simulink model "sampleModel2432_pp_1_2"  (R2018a)
settings: Solver=VariableStepAuto  StartTime=0.0  StopTime=10.0  RelTol=1e-3
undefined symbols (not defined in the file or in its folder): DiscIntNeverNeededParam, sigbuilder_block
libraries: simulink x302
(part 5 of 7)

== system sampleModel2432_pp_1_2/cfblk202/cfblk11 ==
  cfblk1 : Inport
  Action Port : ActionPort  ActionType=else
  cfblk10 : simulink/Discrete/Tapped Delay  vinit=0.0  samptime=-1  NumDelays=1  DelayOrder=Oldest  includeCurrent=off
  cfblk11 : Delay
  cfblk12 : Delay
  cfblk14 : Delay
  cfblk3 : Delay  DelayLengthSource=Input port
      settings: InputPortMap=u0,p1
  cfblk4 : simulink/Continuous/PID Controller (2DOF)  Controller=PID  TimeDomain=Discrete-time  SampleTime=-1  IntegratorMethod=Forward Euler  FilterMethod=Forward Euler  Form=Parallel  UseFilter=on  ControllerParametersSource=internal  P=1  I=1  D=0  N=100  b=1  c=1  InitialConditionSource=internal  InitialConditionForIntegrator=0  InitialConditionForFilter=0  ExternalReset=none  LimitOutput=off  UpperSaturationLimit=inf  LowerSaturationLimit=-inf  LinearizeAsGain=off  AntiWindupMode=none  Kb=1  TrackingMode=off  Kt=1  PParamMin=[]  PParamMax=[]  IParamMin=[]  IParamMax=[]  DParamMin=[]  DParamMax=[]  NParamMin=[]  NParamMax=[]  bParamMin=[]  bParamMax=[]  cParamMin=[]  cParamMax=[]  KbParamMin=[]  KbParamMax=[]  KtParamMin=[]  KtParamMax=[]  POutMin=[]  POutMax=[]  IOutMin=[]  IOutMax=[]  DOutMin=[]  DOutMax=[]  NOutMin=[]  NOutMax=[]  bOutMin=[]  bOutMax=[]  cOutMin=[]  cOutMax=[]  KbOutMin=[]  KbOutMax=[]  KtOutMin=[]  KtOutMax=[]  IntegratorOutMin=[]  IntegratorOutMax=[]  FilterOutMin=[]  FilterOutMax=[]  SumOutMin=[]  SumOutMax=[]  Sum1OutMin=[]  Sum1OutMax=[]  Sum2OutMin=[]  Sum2OutMax=[]  Sum3OutMin=[]  Sum3OutMax=[]  SumI1OutMin=[]  SumI1OutMax=[]  SumI2OutMin=[]  SumI2OutMax=[]  SumI3OutMin=[]  SumI3OutMax=[]  SumDOutMin=[]  SumDOutMax=[]  SaturationOutMin=[]  SaturationOutMax=[]  IntegratorContinuousStateAttributes=''  IntegratorStateMustResolveToSignalObject=off  IntegratorRTWStateStorageClass=Auto  FilterContinuousStateAttributes=''  FilterStateMustResolveToSignalObject=off  FilterRTWStateStorageClass=Auto  DifferentiatorICPrevScaledInput=0  DifferentiatorOutMin=[]  DifferentiatorOutMax=[]  FilterDiffOutCoefMin=[]  FilterDiffOutCoefMax=[]  SumDenOutMin=[]  SumDenOutMax=[]  SumNumOutMin=[]  SumNumOutMax=[]  ReciprocalOutMin=[]  ReciprocalOutMax=[]  DivideOutMin=[]  DivideOutMax=[]  TunerSelectOption=Transfer Function Based (PID Tuner App)
  cfblk5 : simulink/Continuous/PID Controller (2DOF)  Controller=PID  TimeDomain=Discrete-time  SampleTime=-1  IntegratorMethod=Forward Euler  FilterMethod=Forward Euler  Form=Parallel  UseFilter=on  ControllerParametersSource=internal  P=1  I=1  D=0  N=100  b=1  c=1  InitialConditionSource=internal  InitialConditionForIntegrator=0  InitialConditionForFilter=0  ExternalReset=none  LimitOutput=off  UpperSaturationLimit=inf  LowerSaturationLimit=-inf  LinearizeAsGain=off  AntiWindupMode=none  Kb=1  TrackingMode=off  Kt=1  PParamMin=[]  PParamMax=[]  IParamMin=[]  IParamMax=[]  DParamMin=[]  DParamMax=[]  NParamMin=[]  NParamMax=[]  bParamMin=[]  bParamMax=[]  cParamMin=[]  cParamMax=[]  KbParamMin=[]  KbParamMax=[]  KtParamMin=[]  KtParamMax=[]  POutMin=[]  POutMax=[]  IOutMin=[]  IOutMax=[]  DOutMin=[]  DOutMax=[]  NOutMin=[]  NOutMax=[]  bOutMin=[]  bOutMax=[]  cOutMin=[]  cOutMax=[]  KbOutMin=[]  KbOutMax=[]  KtOutMin=[]  KtOutMax=[]  IntegratorOutMin=[]  IntegratorOutMax=[]  FilterOutMin=[]  FilterOutMax=[]  SumOutMin=[]  SumOutMax=[]  Sum1OutMin=[]  Sum1OutMax=[]  Sum2OutMin=[]  Sum2OutMax=[]  Sum3OutMin=[]  Sum3OutMax=[]  SumI1OutMin=[]  SumI1OutMax=[]  SumI2OutMin=[]  SumI2OutMax=[]  SumI3OutMin=[]  SumI3OutMax=[]  SumDOutMin=[]  SumDOutMax=[]  SaturationOutMin=[]  SaturationOutMax=[]  IntegratorContinuousStateAttributes=''  IntegratorStateMustResolveToSignalObject=off  IntegratorRTWStateStorageClass=Auto  FilterContinuousStateAttributes=''  FilterStateMustResolveToSignalObject=off  FilterRTWStateStorageClass=Auto  DifferentiatorICPrevScaledInput=0  DifferentiatorOutMin=[]  DifferentiatorOutMax=[]  FilterDiffOutCoefMin=[]  FilterDiffOutCoefMax=[]  SumDenOutMin=[]  SumDenOutMax=[]  SumNumOutMin=[]  SumNumOutMax=[]  ReciprocalOutMin=[]  ReciprocalOutMax=[]  DivideOutMin=[]  DivideOutMax=[]  TunerSelectOption=Transfer Function Based (PID Tuner App)
  cfblk6 : simulink/Continuous/PID Controller (2DOF)  Controller=PID  TimeDomain=Discrete-time  SampleTime=-1  IntegratorMethod=Forward Euler  FilterMethod=Forward Euler  Form=Parallel  UseFilter=on  ControllerParametersSource=internal  P=1  I=1  D=0  N=100  b=1  c=1  InitialConditionSource=internal  InitialConditionForIntegrator=0  InitialConditionForFilter=0  ExternalReset=none  LimitOutput=off  UpperSaturationLimit=inf  LowerSaturationLimit=-inf  LinearizeAsGain=off  AntiWindupMode=none  Kb=1  TrackingMode=off  Kt=1  PParamMin=[]  PParamMax=[]  IParamMin=[]  IParamMax=[]  DParamMin=[]  DParamMax=[]  NParamMin=[]  NParamMax=[]  bParamMin=[]  bParamMax=[]  cParamMin=[]  cParamMax=[]  KbParamMin=[]  KbParamMax=[]  KtParamMin=[]  KtParamMax=[]  POutMin=[]  POutMax=[]  IOutMin=[]  IOutMax=[]  DOutMin=[]  DOutMax=[]  NOutMin=[]  NOutMax=[]  bOutMin=[]  bOutMax=[]  cOutMin=[]  cOutMax=[]  KbOutMin=[]  KbOutMax=[]  KtOutMin=[]  KtOutMax=[]  IntegratorOutMin=[]  IntegratorOutMax=[]  FilterOutMin=[]  FilterOutMax=[]  SumOutMin=[]  SumOutMax=[]  Sum1OutMin=[]  Sum1OutMax=[]  Sum2OutMin=[]  Sum2OutMax=[]  Sum3OutMin=[]  Sum3OutMax=[]  SumI1OutMin=[]  SumI1OutMax=[]  SumI2OutMin=[]  SumI2OutMax=[]  SumI3OutMin=[]  SumI3OutMax=[]  SumDOutMin=[]  SumDOutMax=[]  SaturationOutMin=[]  SaturationOutMax=[]  IntegratorContinuousStateAttributes=''  IntegratorStateMustResolveToSignalObject=off  IntegratorRTWStateStorageClass=Auto  FilterContinuousStateAttributes=''  FilterStateMustResolveToSignalObject=off  FilterRTWStateStorageClass=Auto  DifferentiatorICPrevScaledInput=0  DifferentiatorOutMin=[]  DifferentiatorOutMax=[]  FilterDiffOutCoefMin=[]  FilterDiffOutCoefMax=[]  SumDenOutMin=[]  SumDenOutMax=[]  SumNumOutMin=[]  SumNumOutMax=[]  ReciprocalOutMin=[]  ReciprocalOutMax=[]  DivideOutMin=[]  DivideOutMax=[]  TunerSelectOption=Transfer Function Based (PID Tuner App)
  cfblk7 : DiscreteTransferFcn
  cfblk8 : DiscreteFilter
  cfblk9 : simulink/Discrete/Transfer Fcn Real Zero  ZeroZ=0.75  ICPrevInput=0.0  DoSatur=off
      settings: SourceProductName=Simulink  SourceProductBaseCode=SL
  cyemi_{239..253} (15 alike) : DataTypeConversion  OutDataTypeStr=double
  cfblk2 : Outport
  cfblk13 : Outport  Port=2
  wires:
  cfblk7/1 -> cyemi_244/1, cyemi_246/1
  cfblk9/1 -> cyemi_241/1, cyemi_242/1
  cfblk10/1 -> cyemi_240/1, cyemi_245/1, cyemi_252/1
  cfblk5/1 -> cfblk2/1, cyemi_253/1
  cfblk6/1 -> cfblk13/1
  cyemi_239/1 -> cfblk10/1
  cfblk1/1 -> cyemi_239/1
  cyemi_240/1 -> cfblk11/1
  cyemi_241/1 -> cfblk12/1
  cyemi_242/1 -> cfblk14/1
  cyemi_243/1 -> cfblk3/1
  cfblk8/1 -> cyemi_243/1
  cyemi_244/1 -> cfblk3/2
  cyemi_245/1 -> cfblk4/1
  cyemi_246/1 -> cfblk4/2
  cyemi_247/1 -> cfblk5/1
  cfblk3/1 -> cyemi_247/1
  cyemi_248/1 -> cfblk5/2
  cfblk14/1 -> cyemi_248/1
  cyemi_249/1 -> cfblk6/1
  cfblk4/1 -> cyemi_249/1
  cyemi_250/1 -> cfblk6/2
  cfblk12/1 -> cyemi_250/1
  cyemi_251/1 -> cfblk7/1
  cfblk11/1 -> cyemi_251/1
  cyemi_252/1 -> cfblk8/1
  cyemi_253/1 -> cfblk9/1

== system sampleModel2432_pp_1_2/cfblk202/cfblk12 ==
  cfblk1 : Inport
  cfblk15 : Inport  Port=2
  Action Port : ActionPort  ActionType=then
  cfblk12 : DiscreteStateSpace  SampleTime=-1
  cfblk14 : DiscreteTransferFcn
  cfblk17 : Delay
  cfblk4 : Delay
  cfblk5 : DiscreteTransferFcn
  cfblk6 : simulink/Discrete/Transfer Fcn Lead or Lag  PoleZ=0.95  ZeroZ=0.75  ICPrevOutput=0.0  ICPrevInput=0.0  DoSatur=off
      settings: SourceProductName=Simulink  SourceProductBaseCode=SL
  cfblk8 : Delay
  cyemi_{256..269} (14 alike) : DataTypeConversion  OutDataTypeStr=double
  cfblk2 : Outport
  cfblk16 : Outport  Port=2
  wires:
  cfblk4/1 -> cyemi_260/1, cyemi_265/1
  cfblk6/1 -> cyemi_256/1
  cfblk15/1 -> cyemi_258/1
  cyemi_259/1 -> cfblk12/1
  cyemi_261/1 -> cfblk14/1
  cfblk8/1 -> cyemi_261/1
  cyemi_262/1 -> cfblk17/1
  cfblk12/1 -> cyemi_262/1
  cfblk17/1 -> cyemi_263/1
  cyemi_264/1 -> cfblk4/1
  cyemi_265/1 -> cfblk5/1
  cyemi_266/1 -> cfblk6/1
  cfblk14/1 -> cyemi_266/1
  cfblk1/1 -> cyemi_267/1
  cyemi_268/1 -> cfblk8/1
  cfblk5/1 -> cyemi_269/1
  cyemi_260/1 -> cfblk2/1
  cyemi_263/1 -> cyemi_268/1
  cyemi_258/1 -> cyemi_264/1
  cyemi_269/1 -> cyemi_257/1
  cyemi_267/1 -> cfblk16/1
  cyemi_256/1 -> cyemi_259/1

== system sampleModel2432_pp_1_2/cfblk202/cfblk13 ==
  cfblk1 : Inport
  cfblk7 : Inport  Port=2
  Action Port : ActionPort  ActionType=else
  cfblk3 : simulink/Discrete/Transfer Fcn Real Zero  ZeroZ=0.75  ICPrevInput=0.0  DoSatur=off
      settings: SourceProductName=Simulink  SourceProductBaseCode=SL
  cfblk4 : Delay  ShowEnablePort=on
      settings: InputPortMap=u0,e6
  cfblk5 : Delay  DelayLengthSource=Input port
      settings: InputPortMap=u0,p1
  cfblk6 : simulink/Discrete/Tapped Delay  vinit=0.0  samptime=-1  NumDelays=1  DelayOrder=Oldest  includeCurrent=off
  cyemi_{272..277} (6 alike) : DataTypeConversion  OutDataTypeStr=double
  cfblk2 : Outport
  wires:
  cfblk4/1 -> cfblk2/1
  cfblk6/1 -> cyemi_274/1, cyemi_276/1
  cyemi_272/1 -> cfblk3/1
  cfblk5/1 -> cyemi_272/1
  cyemi_273/1 -> cfblk4/1
  cfblk3/1 -> cyemi_273/1
  cyemi_274/1 -> cfblk4/2
  cyemi_275/1 -> cfblk5/1
  cfblk7/1 -> cyemi_275/1
  cyemi_276/1 -> cfblk5/2
  cyemi_277/1 -> cfblk6/1
  cfblk1/1 -> cyemi_277/1

== system sampleModel2432_pp_1_2/cfblk204/cfblk13 ==
  cfblk1 : Inport
  cfblk11 : Inport  Port=2
  Action Port : ActionPort  ActionType=then
  cfblk3 : simulink/Discrete/Transfer Fcn Real Zero  ZeroZ=0.75  ICPrevInput=0.0  DoSatur=off
      settings: SourceProductName=Simulink  SourceProductBaseCode=SL
  cfblk4 : simulink/Discrete/Transfer Fcn First Order  PoleZ=0.95  ICPrevOutput=0.0  DoSatur=off
      settings: SourceProductName=Simulink
  cfblk8 : DiscreteStateSpace  SampleTime=-1
  cfblk9 : Delay
  cyemi_{310..317} (8 alike) : DataTypeConversion  OutDataTypeStr=double
  cfblk2 : Outport
  cfblk12 : Outport  Port=2
  wires:
  cfblk9/1 -> cfblk12/1
  cfblk4/1 -> cfblk2/1
  cfblk1/1 -> cyemi_310/1
  cyemi_311/1 -> cfblk3/1
  cyemi_312/1 -> cfblk4/1
  cfblk11/1 -> cyemi_312/1
  cyemi_316/1 -> cfblk8/1
  cfblk3/1 -> cyemi_316/1
  cyemi_317/1 -> cfblk9/1
  cfblk8/1 -> cyemi_317/1
  cyemi_313/1 -> cyemi_311/1
  cyemi_315/1 -> cyemi_314/1
  cyemi_314/1 -> cyemi_313/1
  cyemi_310/1 -> cyemi_315/1

== system sampleModel2432_pp_1_2/cfblk204/cfblk14 ==
  cfblk1 : Inport
  cfblk9 : Inport  Port=2
  Action Port : ActionPort  ActionType=else
  cfblk3 : DiscreteZeroPole  Poles=[0 0.5]  Gain=1  SampleTime=-1
  cfblk4 : UnitDelay  SampleTime=-1
  cfblk5 : simulink/Discrete/Tapped Delay  vinit=0.0  samptime=-1  NumDelays=1  DelayOrder=Oldest  includeCurrent=off
  cfblk6 : UnitDelay  SampleTime=-1
  cfblk7 : DiscreteZeroPole  Poles=[0 0.5]  Gain=1  SampleTime=-1
  cfblk8 : simulink/Discrete/Transfer Fcn First Order  PoleZ=0.95  ICPrevOutput=0.0  DoSatur=off
      settings: SourceProductName=Simulink
  cyemi_{320..325} (6 alike) : DataTypeConversion  OutDataTypeStr=double
  cfblk2 : Outport
  cfblk10 : Outport  Port=2
  cfblk11 : Outport  Port=3
  cfblk12 : Outport  Port=4
  wires:
  cfblk7/1 -> cfblk10/1
  cfblk8/1 -> cfblk12/1
  cfblk3/1 -> cfblk2/1, cyemi_324/1
  cfblk5/1 -> cfblk11/1, cyemi_320/1
  cyemi_320/1 -> cfblk3/1
  cyemi_321/1 -> cfblk4/1
  cfblk1/1 -> cyemi_321/1
  cyemi_322/1 -> cfblk5/1
  cfblk6/1 -> cyemi_322/1
  cyemi_323/1 -> cfblk6/1
  cfblk4/1 -> cyemi_323/1
  cyemi_324/1 -> cfblk7/1
  cyemi_325/1 -> cfblk8/1
  cfblk9/1 -> cyemi_325/1

== system sampleModel2432_pp_1_2/cfblk206/cfblk11 ==
  cfblk1 : Inport
  cfblk8 : Inport  Port=2
  cfblk9 : Inport  Port=3
  Action Port : ActionPort  ActionType=then
  cfblk3 : simulink/Discrete/Difference  ICPrevInput=0.0  OutMin=[]  OutMax=[]  OutDataTypeStr=Inherit: Inherit via back propagation  OutDataType=fixdt(1, 16)  OutScaling=2^-10  DoSatur=off
  cfblk5 : simulink/Discrete/Difference  ICPrevInput=0.0  OutMin=[]  OutMax=[]  OutDataTypeStr=Inherit: Inherit via back propagation  OutDataType=fixdt(1, 16)  OutScaling=2^-10  DoSatur=off
  cfblk6 : simulink/Discrete/Transfer Fcn Real Zero  ZeroZ=0.75  ICPrevInput=0.0  DoSatur=off
      settings: SourceProductName=Simulink  SourceProductBaseCode=SL
  cyemi_{344..348} (5 alike) : DataTypeConversion  OutDataTypeStr=double
  cfblk2 : Outport
  cfblk10 : Outport  Port=2
  wires:
  cfblk9/1 -> cfblk10/1
  cyemi_344/1 -> cfblk3/1
  cfblk6/1 -> cyemi_344/1
  cfblk5/1 -> cyemi_345/1
  cyemi_346/1 -> cfblk5/1
  cfblk8/1 -> cyemi_346/1
  cyemi_347/1 -> cfblk6/1
  cfblk1/1 -> cyemi_347/1
  cyemi_345/1 -> cyemi_348/1
  cyemi_348/1 -> cfblk2/1

== system sampleModel2432_pp_1_2/cfblk206/cfblk12 ==
  cfblk1 : Inport
  cfblk13 : Inport  Port=2
  cfblk14 : Inport  Port=3
  Action Port : ActionPort  ActionType=else
  cfblk10 : simulink/Discrete/Difference  ICPrevInput=0.0  OutMin=[]  OutMax=[]  OutDataTypeStr=Inherit: Inherit via back propagation  OutDataType=fixdt(1, 16)  OutScaling=2^-10  DoSatur=off
  cfblk11 : DiscreteZeroPole  Poles=[0 0.5]  Gain=1  SampleTime=-1
  cfblk12 : UnitDelay  SampleTime=-1
  cfblk16 : Delay
  cfblk3 : DiscreteZeroPole  Poles=[0 0.5]  Gain=1  SampleTime=-1
  cfblk4 : DiscreteFilter
  cfblk5 : DiscreteFilter
  cfblk6 : DiscreteStateSpace  SampleTime=-1
  cfblk7 : DiscreteStateSpace  SampleTime=-1
  cfblk8 : DiscreteTransferFcn
  cfblk9 : DiscreteFilter
  cyemi_{352..362} (11 alike) : DataTypeConversion  OutDataTypeStr=double
  cfblk2 : Outport
  cfblk15 : Outport  Port=2
  wires:
  cfblk10/1 -> cfblk15/1
  cfblk6/1 -> cfblk2/1
  cyemi_352/1 -> cfblk10/1
  cfblk5/1 -> cyemi_352/1
  cyemi_353/1 -> cfblk11/1
  cfblk7/1 -> cyemi_353/1
  cyemi_354/1 -> cfblk12/1
  cfblk13/1 -> cyemi_354/1
  cyemi_355/1 -> cfblk16/1
  cfblk11/1 -> cyemi_355/1
  cyemi_356/1 -> cfblk3/1
  cfblk14/1 -> cyemi_356/1
  cyemi_357/1 -> cfblk4/1
  cfblk16/1 -> cyemi_357/1
  cyemi_358/1 -> cfblk5/1
  cfblk1/1 -> cyemi_358/1
  cyemi_359/1 -> cfblk6/1
  cfblk8/1 -> cyemi_359/1
  cyemi_360/1 -> cfblk7/1
  cfblk9/1 -> cyemi_360/1
  cyemi_361/1 -> cfblk8/1
  cfblk3/1 -> cyemi_361/1
  cyemi_362/1 -> cfblk9/1
  cfblk4/1 -> cyemi_362/1

== system sampleModel2432_pp_1_2/cfblk210/cfblk10 ==
  cfblk1 : Inport
  Action Port : ActionPort  ActionType=then
  cfblk3 : simulink/Discrete/Transfer Fcn First Order  PoleZ=0.95  ICPrevOutput=0.0  DoSatur=off
      settings: SourceProductName=Simulink
  cfblk4 : DiscreteTransferFcn
  cfblk5 : simulink/Discrete/Transfer Fcn Lead or Lag  PoleZ=0.95  ZeroZ=0.75  ICPrevOutput=0.0  ICPrevInput=0.0  DoSatur=off
      settings: SourceProductName=Simulink  SourceProductBaseCode=SL
  cfblk9 : Delay
  cyemi_{399..404} (6 alike) : DataTypeConversion  OutDataTypeStr=double
  cfblk2 : Outport
  cfblk7 : Outport  Port=2
  cfblk8 : Outport  Port=3
  wires:
  cfblk5/1 -> cfblk8/1, cyemi_404/1
  cfblk4/1 -> cfblk2/1, cyemi_401/1
  cfblk1/1 -> cfblk7/1, cyemi_403/1
  cyemi_399/1 -> cfblk3/1
  cyemi_400/1 -> cfblk4/1
  cfblk3/1 -> cyemi_400/1
  cyemi_401/1 -> cfblk5/1
  cfblk9/1 -> cyemi_402/1
  cyemi_404/1 -> cfblk9/1
  cyemi_402/1 -> cyemi_399/1

== system sampleModel2432_pp_1_2/cfblk210/cfblk11 ==
  cfblk1 : Inport
  cfblk12 : Inport  Port=2
  Action Port : ActionPort  ActionType=else
  cfblk10 : DiscreteStateSpace  SampleTime=-1
  cfblk11 : DiscreteStateSpace  SampleTime=-1
  cfblk15 : Delay
  cfblk3 : simulink/Continuous/PID Controller (2DOF)  Controller=PID  TimeDomain=Discrete-time  SampleTime=-1  IntegratorMethod=Forward Euler  FilterMethod=Forward Euler  Form=Parallel  UseFilter=on  ControllerParametersSource=internal  P=1  I=1  D=0  N=100  b=1  c=1  InitialConditionSource=internal  InitialConditionForIntegrator=0  InitialConditionForFilter=0  ExternalReset=none  LimitOutput=off  UpperSaturationLimit=inf  LowerSaturationLimit=-inf  LinearizeAsGain=off  AntiWindupMode=none  Kb=1  TrackingMode=off  Kt=1  PParamMin=[]  PParamMax=[]  IParamMin=[]  IParamMax=[]  DParamMin=[]  DParamMax=[]  NParamMin=[]  NParamMax=[]  bParamMin=[]  bParamMax=[]  cParamMin=[]  cParamMax=[]  KbParamMin=[]  KbParamMax=[]  KtParamMin=[]  KtParamMax=[]  POutMin=[]  POutMax=[]  IOutMin=[]  IOutMax=[]  DOutMin=[]  DOutMax=[]  NOutMin=[]  NOutMax=[]  bOutMin=[]  bOutMax=[]  cOutMin=[]  cOutMax=[]  KbOutMin=[]  KbOutMax=[]  KtOutMin=[]  KtOutMax=[]  IntegratorOutMin=[]  IntegratorOutMax=[]  FilterOutMin=[]  FilterOutMax=[]  SumOutMin=[]  SumOutMax=[]  Sum1OutMin=[]  Sum1OutMax=[]  Sum2OutMin=[]  Sum2OutMax=[]  Sum3OutMin=[]  Sum3OutMax=[]  SumI1OutMin=[]  SumI1OutMax=[]  SumI2OutMin=[]  SumI2OutMax=[]  SumI3OutMin=[]  SumI3OutMax=[]  SumDOutMin=[]  SumDOutMax=[]  SaturationOutMin=[]  SaturationOutMax=[]  IntegratorContinuousStateAttributes=''  IntegratorStateMustResolveToSignalObject=off  IntegratorRTWStateStorageClass=Auto  FilterContinuousStateAttributes=''  FilterStateMustResolveToSignalObject=off  FilterRTWStateStorageClass=Auto  DifferentiatorICPrevScaledInput=0  DifferentiatorOutMin=[]  DifferentiatorOutMax=[]  FilterDiffOutCoefMin=[]  FilterDiffOutCoefMax=[]  SumDenOutMin=[]  SumDenOutMax=[]  SumNumOutMin=[]  SumNumOutMax=[]  ReciprocalOutMin=[]  ReciprocalOutMax=[]  DivideOutMin=[]  DivideOutMax=[]  TunerSelectOption=Transfer Function Based (PID Tuner App)
  cfblk4 : DiscreteZeroPole  Poles=[0 0.5]  Gain=1  SampleTime=-1
  cfblk5 : simulink/Discrete/Transfer Fcn Real Zero  ZeroZ=0.75  ICPrevInput=0.0  DoSatur=off
      settings: SourceProductName=Simulink  SourceProductBaseCode=SL
  cfblk6 : Delay  ShowEnablePort=on
      settings: InputPortMap=u0,e6
  cfblk7 : simulink/Continuous/PID Controller (2DOF)  Controller=PID  TimeDomain=Discrete-time  SampleTime=-1  IntegratorMethod=Forward Euler  FilterMethod=Forward Euler  Form=Parallel  UseFilter=on  ControllerParametersSource=internal  P=1  I=1  D=0  N=100  b=1  c=1  InitialConditionSource=internal  InitialConditionForIntegrator=0  InitialConditionForFilter=0  ExternalReset=none  LimitOutput=off  UpperSaturationLimit=inf  LowerSaturationLimit=-inf  LinearizeAsGain=off  AntiWindupMode=none  Kb=1  TrackingMode=off  Kt=1  PParamMin=[]  PParamMax=[]  IParamMin=[]  IParamMax=[]  DParamMin=[]  DParamMax=[]  NParamMin=[]  NParamMax=[]  bParamMin=[]  bParamMax=[]  cParamMin=[]  cParamMax=[]  KbParamMin=[]  KbParamMax=[]  KtParamMin=[]  KtParamMax=[]  POutMin=[]  POutMax=[]  IOutMin=[]  IOutMax=[]  DOutMin=[]  DOutMax=[]  NOutMin=[]  NOutMax=[]  bOutMin=[]  bOutMax=[]  cOutMin=[]  cOutMax=[]  KbOutMin=[]  KbOutMax=[]  KtOutMin=[]  KtOutMax=[]  IntegratorOutMin=[]  IntegratorOutMax=[]  FilterOutMin=[]  FilterOutMax=[]  SumOutMin=[]  SumOutMax=[]  Sum1OutMin=[]  Sum1OutMax=[]  Sum2OutMin=[]  Sum2OutMax=[]  Sum3OutMin=[]  Sum3OutMax=[]  SumI1OutMin=[]  SumI1OutMax=[]  SumI2OutMin=[]  SumI2OutMax=[]  SumI3OutMin=[]  SumI3OutMax=[]  SumDOutMin=[]  SumDOutMax=[]  SaturationOutMin=[]  SaturationOutMax=[]  IntegratorContinuousStateAttributes=''  IntegratorStateMustResolveToSignalObject=off  IntegratorRTWStateStorageClass=Auto  FilterContinuousStateAttributes=''  FilterStateMustResolveToSignalObject=off  FilterRTWStateStorageClass=Auto  DifferentiatorICPrevScaledInput=0  DifferentiatorOutMin=[]  DifferentiatorOutMax=[]  FilterDiffOutCoefMin=[]  FilterDiffOutCoefMax=[]  SumDenOutMin=[]  SumDenOutMax=[]  SumNumOutMin=[]  SumNumOutMax=[]  ReciprocalOutMin=[]  ReciprocalOutMax=[]  DivideOutMin=[]  DivideOutMax=[]  TunerSelectOption=Transfer Function Based (PID Tuner App)
  cfblk8 : DiscreteFir
  cfblk9 : DiscreteZeroPole  Poles=[0 0.5]  Gain=1  SampleTime=-1
  cyemi_{407..419} (13 alike) : DataTypeConversion  OutDataTypeStr=double
  cfblk2 : Outport
  cfblk13 : Outport  Port=2
  cfblk14 : Outport  Port=3
  wires:
  cfblk8/1 -> cfblk2/1, cyemi_408/1
  cfblk11/1 -> cyemi_407/1, cyemi_414/1
  cfblk7/1 -> cfblk13/1
  cfblk3/1 -> cfblk14/1, cyemi_415/1
  cyemi_407/1 -> cfblk10/1
  cyemi_408/1 -> cfblk11/1
  cyemi_409/1 -> cfblk15/1
  cfblk10/1 -> cyemi_409/1
  cyemi_410/1 -> cfblk3/1
  cfblk12/1 -> cyemi_410/1
  cyemi_411/1 -> cfblk3/2
  cfblk4/1 -> cyemi_411/1
  cyemi_412/1 -> cfblk4/1
  cfblk9/1 -> cyemi_412/1
  cyemi_413/1 -> cfblk5/1
  cfblk15/1 -> cyemi_413/1
  cyemi_414/1 -> cfblk6/1
  cyemi_415/1 -> cfblk6/2
  cyemi_416/1 -> cfblk7/1
  cfblk6/1 -> cyemi_416/1, cyemi_417/1
  cyemi_417/1 -> cfblk7/2
  cyemi_418/1 -> cfblk8/1
  cfblk5/1 -> cyemi_418/1
  cyemi_419/1 -> cfblk9/1
  cfblk1/1 -> cyemi_419/1

== system sampleModel2432_pp_1_2/cfblk218/cfblk18 ==
  cfblk1 : Inport
  cfblk11 : Inport  Port=2
  Action Port : ActionPort  ActionType=then
  cfblk10 : simulink/Discrete/Transfer Fcn First Order  PoleZ=0.95  ICPrevOutput=0.0  DoSatur=off
      settings: SourceProductName=Simulink
  cfblk5 : DiscreteStateSpace  SampleTime=-1
  cfblk6 : Delay
  cfblk7 : simulink/Discrete/Transfer Fcn Lead or Lag  PoleZ=0.95  ZeroZ=0.75  ICPrevOutput=0.0  ICPrevInput=0.0  DoSatur=off
      settings: SourceProductName=Simulink  SourceProductBaseCode=SL
  cfblk9 : DiscreteFir
  cyemi_{505..512} (8 alike) : DataTypeConversion  OutDataTypeStr=double
  cfblk2 : Outport
  cfblk12 : Outport  Port=2
  cfblk13 : Outport  Port=3
  wires:
  cfblk7/1 -> cfblk13/1
  cfblk1/1 -> cfblk12/1
  cfblk11/1 -> cyemi_510/1, cyemi_511/1
  cyemi_505/1 -> cfblk10/1
  cfblk9/1 -> cyemi_505/1
  cfblk5/1 -> cyemi_506/1
  cfblk10/1 -> cyemi_507/1
  cyemi_508/1 -> cfblk5/1
  cfblk6/1 -> cyemi_508/1
  cyemi_509/1 -> cfblk6/1
  cyemi_510/1 -> cfblk7/1
  cyemi_512/1 -> cfblk9/1
  cyemi_507/1 -> cyemi_509/1
  cyemi_511/1 -> cyemi_512/1
  cyemi_506/1 -> cfblk2/1

== system sampleModel2432_pp_1_2/cfblk218/cfblk19 ==
  cfblk1 : Inport
  cfblk10 : Inport  Port=2
  Action Port : ActionPort  ActionType=else
  cfblk11 : Delay
  cfblk3 : simulink/Discrete/Tapped Delay  vinit=0.0  samptime=-1  NumDelays=1  DelayOrder=Oldest  includeCurrent=off
  cfblk4 : Delay
  cfblk5 : Delay  ShowEnablePort=on
      settings: InputPortMap=u0,e6
  cfblk6 : DiscreteZeroPole  Poles=[0 0.5]  Gain=1  SampleTime=-1
  cfblk7 : simulink/Continuous/PID Controller (2DOF)  Controller=PID  TimeDomain=Discrete-time  SampleTime=-1  IntegratorMethod=Forward Euler  FilterMethod=Forward Euler  Form=Parallel  UseFilter=on  ControllerParametersSource=internal  P=1  I=1  D=0  N=100  b=1  c=1  InitialConditionSource=internal  InitialConditionForIntegrator=0  InitialConditionForFilter=0  ExternalReset=none  LimitOutput=off  UpperSaturationLimit=inf  LowerSaturationLimit=-inf  LinearizeAsGain=off  AntiWindupMode=none  Kb=1  TrackingMode=off  Kt=1  PParamMin=[]  PParamMax=[]  IParamMin=[]  IParamMax=[]  DParamMin=[]  DParamMax=[]  NParamMin=[]  NParamMax=[]  bParamMin=[]  bParamMax=[]  cParamMin=[]  cParamMax=[]  KbParamMin=[]  KbParamMax=[]  KtParamMin=[]  KtParamMax=[]  POutMin=[]  POutMax=[]  IOutMin=[]  IOutMax=[]  DOutMin=[]  DOutMax=[]  NOutMin=[]  NOutMax=[]  bOutMin=[]  bOutMax=[]  cOutMin=[]  cOutMax=[]  KbOutMin=[]  KbOutMax=[]  KtOutMin=[]  KtOutMax=[]  IntegratorOutMin=[]  IntegratorOutMax=[]  FilterOutMin=[]  FilterOutMax=[]  SumOutMin=[]  SumOutMax=[]  Sum1OutMin=[]  Sum1OutMax=[]  Sum2OutMin=[]  Sum2OutMax=[]  Sum3OutMin=[]  Sum3OutMax=[]  SumI1OutMin=[]  SumI1OutMax=[]  SumI2OutMin=[]  SumI2OutMax=[]  SumI3OutMin=[]  SumI3OutMax=[]  SumDOutMin=[]  SumDOutMax=[]  SaturationOutMin=[]  SaturationOutMax=[]  IntegratorContinuousStateAttributes=''  IntegratorStateMustResolveToSignalObject=off  IntegratorRTWStateStorageClass=Auto  FilterContinuousStateAttributes=''  FilterStateMustResolveToSignalObject=off  FilterRTWStateStorageClass=Auto  DifferentiatorICPrevScaledInput=0  DifferentiatorOutMin=[]  DifferentiatorOutMax=[]  FilterDiffOutCoefMin=[]  FilterDiffOutCoefMax=[]  SumDenOutMin=[]  SumDenOutMax=[]  SumNumOutMin=[]  SumNumOutMax=[]  ReciprocalOutMin=[]  ReciprocalOutMax=[]  DivideOutMin=[]  DivideOutMax=[]  TunerSelectOption=Transfer Function Based (PID Tuner App)
  cfblk8 : simulink/Discrete/Difference  ICPrevInput=0.0  OutMin=[]  OutMax=[]  OutDataTypeStr=Inherit: Inherit via back propagation  OutDataType=fixdt(1, 16)  OutScaling=2^-10  DoSatur=off
  cfblk9 : simulink/Discrete/Difference  ICPrevInput=0.0  OutMin=[]  OutMax=[]  OutDataTypeStr=Inherit: Inherit via back propagation  OutDataType=fixdt(1, 16)  OutScaling=2^-10  DoSatur=off
  cyemi_{515..524} (10 alike) : DataTypeConversion  OutDataTypeStr=double
  cfblk2 : Outport
  wires:
  cfblk6/1 -> cfblk2/1
  cfblk10/1 -> cyemi_520/1, cyemi_522/1
  cyemi_515/1 -> cfblk11/1
  cfblk4/1 -> cyemi_515/1
  cyemi_516/1 -> cfblk3/1
  cfblk8/1 -> cyemi_516/1
  cyemi_517/1 -> cfblk4/1
  cfblk5/1 -> cyemi_517/1
  cyemi_518/1 -> cfblk5/1
  cfblk11/1 -> cyemi_518/1
  cyemi_519/1 -> cfblk5/2
  cfblk3/1 -> cyemi_519/1
  cyemi_520/1 -> cfblk6/1
  cyemi_521/1 -> cfblk7/1
  cfblk1/1 -> cyemi_521/1
  cyemi_522/1 -> cfblk7/2
  cyemi_523/1 -> cfblk8/1
  cfblk9/1 -> cyemi_523/1
  cyemi_524/1 -> cfblk9/1
  cfblk7/1 -> cyemi_524/1

== system sampleModel2432_pp_1_2/cfblk218/cfblk20 ==
  cfblk1 : Inport
  cfblk10 : Inport  Port=2
  Action Port : ActionPort  ActionType=then
  cfblk3 : DiscreteIntegrator  SampleTime=-1  ICPrevOutput=DiscIntNeverNeededParam  ICPrevScaledInput=DiscIntNeverNeededParam
  cfblk4 : simulink/Discrete/Transfer Fcn Real Zero  ZeroZ=0.75  ICPrevInput=0.0  DoSatur=off
      settings: SourceProductName=Simulink  SourceProductBaseCode=SL
  cfblk6 : DiscreteTransferFcn
  cfblk7 : DiscreteIntegrator  SampleTime=-1  ICPrevOutput=DiscIntNeverNeededParam  ICPrevScaledInput=DiscIntNeverNeededParam
  cfblk9 : DiscreteIntegrator  SampleTime=-1  ICPrevOutput=DiscIntNeverNeededParam  ICPrevScaledInput=DiscIntNeverNeededParam
  cyemi_{527..533} (7 alike) : DataTypeConversion  OutDataTypeStr=double
  cfblk2 : Outport
  cfblk11 : Outport  Port=2
  cfblk12 : Outport  Port=3
  cfblk13 : Outport  Port=4
  cfblk14 : Outport  Port=5
  cfblk15 : Outport  Port=6
  wires:
  cfblk9/1 -> cfblk13/1
  cfblk4/1 -> cfblk14/1
  cfblk6/1 -> cfblk12/1, cfblk2/1, cyemi_529/1
  cfblk3/1 -> cfblk15/1, cyemi_533/1
  cyemi_527/1 -> cfblk3/1
  cfblk10/1 -> cyemi_527/1
  cyemi_528/1 -> cfblk4/1
  cfblk7/1 -> cyemi_528/1
  cyemi_530/1 -> cfblk6/1
  cfblk1/1 -> cyemi_530/1
  cyemi_531/1 -> cfblk7/1
  cyemi_533/1 -> cfblk9/1
  cyemi_532/1 -> cyemi_531/1
  cyemi_529/1 -> cyemi_532/1, cfblk11/1

== system sampleModel2432_pp_1_2/cfblk218/cfblk21 ==
  cfblk1 : Inport
  cfblk6 : Inport  Port=2
  Action Port : ActionPort  ActionType=else
  cfblk3 : simulink/Continuous/PID Controller (2DOF)  Controller=PID  TimeDomain=Discrete-time  SampleTime=-1  IntegratorMethod=Forward Euler  FilterMethod=Forward Euler  Form=Parallel  UseFilter=on  ControllerParametersSource=internal  P=1  I=1  D=0  N=100  b=1  c=1  InitialConditionSource=internal  InitialConditionForIntegrator=0  InitialConditionForFilter=0  ExternalReset=none  LimitOutput=off  UpperSaturationLimit=inf  LowerSaturationLimit=-inf  LinearizeAsGain=off  AntiWindupMode=none  Kb=1  TrackingMode=off  Kt=1  PParamMin=[]  PParamMax=[]  IParamMin=[]  IParamMax=[]  DParamMin=[]  DParamMax=[]  NParamMin=[]  NParamMax=[]  bParamMin=[]  bParamMax=[]  cParamMin=[]  cParamMax=[]  KbParamMin=[]  KbParamMax=[]  KtParamMin=[]  KtParamMax=[]  POutMin=[]  POutMax=[]  IOutMin=[]  IOutMax=[]  DOutMin=[]  DOutMax=[]  NOutMin=[]  NOutMax=[]  bOutMin=[]  bOutMax=[]  cOutMin=[]  cOutMax=[]  KbOutMin=[]  KbOutMax=[]  KtOutMin=[]  KtOutMax=[]  IntegratorOutMin=[]  IntegratorOutMax=[]  FilterOutMin=[]  FilterOutMax=[]  SumOutMin=[]  SumOutMax=[]  Sum1OutMin=[]  Sum1OutMax=[]  Sum2OutMin=[]  Sum2OutMax=[]  Sum3OutMin=[]  Sum3OutMax=[]  SumI1OutMin=[]  SumI1OutMax=[]  SumI2OutMin=[]  SumI2OutMax=[]  SumI3OutMin=[]  SumI3OutMax=[]  SumDOutMin=[]  SumDOutMax=[]  SaturationOutMin=[]  SaturationOutMax=[]  IntegratorContinuousStateAttributes=''  IntegratorStateMustResolveToSignalObject=off  IntegratorRTWStateStorageClass=Auto  FilterContinuousStateAttributes=''  FilterStateMustResolveToSignalObject=off  FilterRTWStateStorageClass=Auto  DifferentiatorICPrevScaledInput=0  DifferentiatorOutMin=[]  DifferentiatorOutMax=[]  FilterDiffOutCoefMin=[]  FilterDiffOutCoefMax=[]  SumDenOutMin=[]  SumDenOutMax=[]  SumNumOutMin=[]  SumNumOutMax=[]  ReciprocalOutMin=[]  ReciprocalOutMax=[]  DivideOutMin=[]  DivideOutMax=[]  TunerSelectOption=Transfer Function Based (PID Tuner App)
  cfblk4 : UnitDelay  SampleTime=-1
  cfblk5 : simulink/Discrete/Difference  ICPrevInput=0.0  OutMin=[]  OutMax=[]  OutDataTypeStr=Inherit: Inherit via back propagation  OutDataType=fixdt(1, 16)  OutScaling=2^-10  DoSatur=off
  cyemi_{536..539} (4 alike) : DataTypeConversion  OutDataTypeStr=double
  cfblk2 : Outport
  cfblk7 : Outport  Port=2
  cfblk8 : Outport  Port=3
  wires:
  cfblk1/1 -> cfblk7/1, cyemi_537/1
  cfblk5/1 -> cfblk8/1, cfblk2/1
  cyemi_536/1 -> cfblk3/1
  cfblk6/1 -> cyemi_536/1
  cyemi_537/1 -> cfblk3/2
  cyemi_538/1 -> cfblk4/1
  cfblk3/1 -> cyemi_538/1
  cyemi_539/1 -> cfblk5/1
  cfblk4/1 -> cyemi_539/1

== system sampleModel2432_pp_1_2/cfblk218/cfblk22 ==
  cfblk1 : Inport
  Action Port : ActionPort  ActionType=then
  cfblk11 : simulink/Discrete/Tapped Delay  vinit=0.0  samptime=-1  NumDelays=1  DelayOrder=Oldest  includeCurrent=off
  cfblk12 : Delay  ShowEnablePort=on
      settings: InputPortMap=u0,e6
  cfblk13 : simulink/Discrete/Transfer Fcn Real Zero  ZeroZ=0.75  ICPrevInput=0.0  DoSatur=off
      settings: SourceProductName=Simulink  SourceProductBaseCode=SL
  cfblk14 : Delay
  cfblk3 : DiscreteIntegrator  SampleTime=-1  ICPrevOutput=DiscIntNeverNeededParam  ICPrevScaledInput=DiscIntNeverNeededParam
  cfblk5 : DiscreteStateSpace  SampleTime=-1
  cfblk7 : DiscreteFilter
  cfblk8 : simulink/Continuous/PID Controller (2DOF)  Controller=PID  TimeDomain=Discrete-time  SampleTime=-1  IntegratorMethod=Forward Euler  FilterMethod=Forward Euler  Form=Parallel  UseFilter=on  ControllerParametersSource=internal  P=1  I=1  D=0  N=100  b=1  c=1  InitialConditionSource=internal  InitialConditionForIntegrator=0  InitialConditionForFilter=0  ExternalReset=none  LimitOutput=off  UpperSaturationLimit=inf  LowerSaturationLimit=-inf  LinearizeAsGain=off  AntiWindupMode=none  Kb=1  TrackingMode=off  Kt=1  PParamMin=[]  PParamMax=[]  IParamMin=[]  IParamMax=[]  DParamMin=[]  DParamMax=[]  NParamMin=[]  NParamMax=[]  bParamMin=[]  bParamMax=[]  cParamMin=[]  cParamMax=[]  KbParamMin=[]  KbParamMax=[]  KtParamMin=[]  KtParamMax=[]  POutMin=[]  POutMax=[]  IOutMin=[]  IOutMax=[]  DOutMin=[]  DOutMax=[]  NOutMin=[]  NOutMax=[]  bOutMin=[]  bOutMax=[]  cOutMin=[]  cOutMax=[]  KbOutMin=[]  KbOutMax=[]  KtOutMin=[]  KtOutMax=[]  IntegratorOutMin=[]  IntegratorOutMax=[]  FilterOutMin=[]  FilterOutMax=[]  SumOutMin=[]  SumOutMax=[]  Sum1OutMin=[]  Sum1OutMax=[]  Sum2OutMin=[]  Sum2OutMax=[]  Sum3OutMin=[]  Sum3OutMax=[]  SumI1OutMin=[]  SumI1OutMax=[]  SumI2OutMin=[]  SumI2OutMax=[]  SumI3OutMin=[]  SumI3OutMax=[]  SumDOutMin=[]  SumDOutMax=[]  SaturationOutMin=[]  SaturationOutMax=[]  IntegratorContinuousStateAttributes=''  IntegratorStateMustResolveToSignalObject=off  IntegratorRTWStateStorageClass=Auto  FilterContinuousStateAttributes=''  FilterStateMustResolveToSignalObject=off  FilterRTWStateStorageClass=Auto  DifferentiatorICPrevScaledInput=0  DifferentiatorOutMin=[]  DifferentiatorOutMax=[]  FilterDiffOutCoefMin=[]  FilterDiffOutCoefMax=[]  SumDenOutMin=[]  SumDenOutMax=[]  SumNumOutMin=[]  SumNumOutMax=[]  ReciprocalOutMin=[]  ReciprocalOutMax=[]  DivideOutMin=[]  DivideOutMax=[]  TunerSelectOption=Transfer Function Based (PID Tuner App)
  cfblk9 : DiscreteIntegrator  SampleTime=-1  ICPrevOutput=DiscIntNeverNeededParam  ICPrevScaledInput=DiscIntNeverNeededParam
  cyemi_{541..554} (14 alike) : DataTypeConversion  OutDataTypeStr=double
  cfblk2 : Outport
  wires:
  cfblk1/1 -> cyemi_549/1, cyemi_554/1
  cfblk7/1 -> cyemi_541/1
  cyemi_542/1 -> cfblk11/1
  cyemi_543/1 -> cfblk12/1
  cfblk11/1 -> cyemi_543/1
  cyemi_544/1 -> cfblk12/2
  cfblk14/1 -> cyemi_544/1
  cyemi_545/1 -> cfblk13/1
  cfblk5/1 -> cyemi_545/1
  cyemi_546/1 -> cfblk14/1
  cfblk3/1 -> cyemi_546/1
  cyemi_547/1 -> cfblk3/1
  cfblk8/1 -> cyemi_547/1
  cfblk12/1 -> cyemi_548/1
  cyemi_549/1 -> cfblk5/1
  cfblk9/1 -> cyemi_550/1
  cyemi_551/1 -> cfblk7/1
  cfblk13/1 -> cyemi_551/1
  cyemi_552/1 -> cfblk8/1
  cyemi_553/1 -> cfblk8/2
  cyemi_554/1 -> cfblk9/1
  cyemi_548/1 -> cyemi_553/1, cyemi_552/1
  cyemi_550/1 -> cyemi_542/1
  cyemi_541/1 -> cfblk2/1

== system sampleModel2432_pp_1_2/cfblk218/cfblk23 ==
  cfblk1 : Inport
  cfblk12 : Inport  Port=2
  cfblk13 : Inport  Port=3
  Action Port : ActionPort  ActionType=else
  cfblk{10,15..17} (4 alike) : Delay
  cfblk11 : DiscreteFir
  cfblk3 : simulink/Continuous/PID Controller (2DOF)  Controller=PID  TimeDomain=Discrete-time  SampleTime=-1  IntegratorMethod=Forward Euler  FilterMethod=Forward Euler  Form=Parallel  UseFilter=on  ControllerParametersSource=internal  P=1  I=1  D=0  N=100  b=1  c=1  InitialConditionSource=internal  InitialConditionForIntegrator=0  InitialConditionForFilter=0  ExternalReset=none  LimitOutput=off  UpperSaturationLimit=inf  LowerSaturationLimit=-inf  LinearizeAsGain=off  AntiWindupMode=none  Kb=1  TrackingMode=off  Kt=1  PParamMin=[]  PParamMax=[]  IParamMin=[]  IParamMax=[]  DParamMin=[]  DParamMax=[]  NParamMin=[]  NParamMax=[]  bParamMin=[]  bParamMax=[]  cParamMin=[]  cParamMax=[]  KbParamMin=[]  KbParamMax=[]  KtParamMin=[]  KtParamMax=[]  POutMin=[]  POutMax=[]  IOutMin=[]  IOutMax=[]  DOutMin=[]  DOutMax=[]  NOutMin=[]  NOutMax=[]  bOutMin=[]  bOutMax=[]  cOutMin=[]  cOutMax=[]  KbOutMin=[]  KbOutMax=[]  KtOutMin=[]  KtOutMax=[]  IntegratorOutMin=[]  IntegratorOutMax=[]  FilterOutMin=[]  FilterOutMax=[]  SumOutMin=[]  SumOutMax=[]  Sum1OutMin=[]  Sum1OutMax=[]  Sum2OutMin=[]  Sum2OutMax=[]  Sum3OutMin=[]  Sum3OutMax=[]  SumI1OutMin=[]  SumI1OutMax=[]  SumI2OutMin=[]  SumI2OutMax=[]  SumI3OutMin=[]  SumI3OutMax=[]  SumDOutMin=[]  SumDOutMax=[]  SaturationOutMin=[]  SaturationOutMax=[]  IntegratorContinuousStateAttributes=''  IntegratorStateMustResolveToSignalObject=off  IntegratorRTWStateStorageClass=Auto  FilterContinuousStateAttributes=''  FilterStateMustResolveToSignalObject=off  FilterRTWStateStorageClass=Auto  DifferentiatorICPrevScaledInput=0  DifferentiatorOutMin=[]  DifferentiatorOutMax=[]  FilterDiffOutCoefMin=[]  FilterDiffOutCoefMax=[]  SumDenOutMin=[]  SumDenOutMax=[]  SumNumOutMin=[]  SumNumOutMax=[]  ReciprocalOutMin=[]  ReciprocalOutMax=[]  DivideOutMin=[]  DivideOutMax=[]  TunerSelectOption=Transfer Function Based (PID Tuner App)
  cfblk4 : UnitDelay  SampleTime=-1
  cfblk5 : simulink/Discrete/Transfer Fcn Real Zero  ZeroZ=0.75  ICPrevInput=0.0  DoSatur=off
      settings: SourceProductName=Simulink  SourceProductBaseCode=SL
  cfblk6 : DiscreteFir
  cfblk7 : Delay  DelayLengthSource=Input port
      settings: InputPortMap=u0,p1
  cfblk8 : Delay  ShowEnablePort=on
      settings: InputPortMap=u0,e6
  cfblk9 : simulink/Discrete/Difference  ICPrevInput=0.0  OutMin=[]  OutMax=[]  OutDataTypeStr=Inherit: Inherit via back propagation  OutDataType=fixdt(1, 16)  OutScaling=2^-10  DoSatur=off
  cyemi_{558..572} (15 alike) : DataTypeConversion  OutDataTypeStr=double
  cfblk2 : Outport
  cfblk14 : Outport  Port=2
  wires:
  cfblk1/1 -> cfblk2/1
  cfblk9/1 -> cyemi_561/1, cyemi_562/1, cyemi_563/1
  cfblk8/1 -> cfblk14/1
  cyemi_558/1 -> cfblk10/1
  cfblk6/1 -> cyemi_558/1
  cyemi_559/1 -> cfblk11/1
  cfblk3/1 -> cyemi_559/1
  cyemi_560/1 -> cfblk15/1
  cfblk4/1 -> cyemi_560/1
  cyemi_561/1 -> cfblk16/1
  cyemi_562/1 -> cfblk17/1
  cyemi_563/1 -> cfblk3/1
  cyemi_564/1 -> cfblk3/2
  cfblk15/1 -> cyemi_564/1
  cyemi_565/1 -> cfblk4/1
  cfblk11/1 -> cyemi_565/1
  cyemi_566/1 -> cfblk5/1
  cfblk10/1 -> cyemi_566/1
  cyemi_567/1 -> cfblk6/1
  cfblk12/1 -> cyemi_567/1
  cyemi_568/1 -> cfblk7/1
  cfblk16/1 -> cyemi_568/1
  cyemi_569/1 -> cfblk7/2
  cfblk17/1 -> cyemi_569/1
  cyemi_570/1 -> cfblk8/1
  cfblk5/1 -> cyemi_570/1
  cyemi_571/1 -> cfblk8/2
  cfblk13/1 -> cyemi_571/1
  cyemi_572/1 -> cfblk9/1
  cfblk7/1 -> cyemi_572/1

== system sampleModel2432_pp_1_2/cfblk219/cfblk10 ==
  cfblk1 : Inport
  Action Port : ActionPort
  cfblk10 : DiscreteStateSpace  SampleTime=-1
  cfblk11 : simulink/Discrete/Difference  ICPrevInput=0.0  OutMin=[]  OutMax=[]  OutDataTypeStr=Inherit: Inherit via back propagation  OutDataType=fixdt(1, 16)  OutScaling=2^-10  DoSatur=off
  cfblk12 : simulink/Continuous/PID Controller  Controller=PID  TimeDomain=Discrete-time  SampleTime=-1  IntegratorMethod=Forward Euler  FilterMethod=Forward Euler  Form=Parallel  UseFilter=on  ControllerParametersSource=internal  P=1  I=1  D=0  N=100  InitialConditionSource=internal  InitialConditionForIntegrator=0  InitialConditionForFilter=0  ExternalReset=none  LimitOutput=off  UpperSaturationLimit=inf  LowerSaturationLimit=-inf  LinearizeAsGain=off  AntiWindupMode=none  Kb=1  TrackingMode=off  Kt=1  PParamMin=[]  PParamMax=[]  IParamMin=[]  IParamMax=[]  DParamMin=[]  DParamMax=[]  NParamMin=[]  NParamMax=[]  KbParamMin=[]  KbParamMax=[]  KtParamMin=[]  KtParamMax=[]  POutMin=[]  POutMax=[]  IOutMin=[]  IOutMax=[]  DOutMin=[]  DOutMax=[]  NOutMin=[]  NOutMax=[]  KbOutMin=[]  KbOutMax=[]  KtOutMin=[]  KtOutMax=[]  IntegratorOutMin=[]  IntegratorOutMax=[]  FilterOutMin=[]  FilterOutMax=[]  SumOutMin=[]  SumOutMax=[]  SumI1OutMin=[]  SumI1OutMax=[]  SumI2OutMin=[]  SumI2OutMax=[]  SumI3OutMin=[]  SumI3OutMax=[]  SumDOutMin=[]  SumDOutMax=[]  SaturationOutMin=[]  SaturationOutMax=[]  IntegratorContinuousStateAttributes=''  IntegratorStateMustResolveToSignalObject=off  IntegratorRTWStateStorageClass=Auto  FilterContinuousStateAttributes=''  FilterStateMustResolveToSignalObject=off  FilterRTWStateStorageClass=Auto  DifferentiatorICPrevScaledInput=0  DifferentiatorOutMin=[]  DifferentiatorOutMax=[]  FilterDiffOutCoefMin=[]  FilterDiffOutCoefMax=[]  SumDenOutMin=[]  SumDenOutMax=[]  SumNumOutMin=[]  SumNumOutMax=[]  ReciprocalOutMin=[]  ReciprocalOutMax=[]  DivideOutMin=[]  DivideOutMax=[]  TunerSelectOption=Transfer Function Based (PID Tuner App)
  cfblk13 : Delay
  cfblk14 : Delay
  cfblk5 : DiscreteFilter
  cfblk7 : simulink/Continuous/PID Controller (2DOF)  Controller=PID  TimeDomain=Discrete-time  SampleTime=-1  IntegratorMethod=Forward Euler  FilterMethod=Forward Euler  Form=Parallel  UseFilter=on  ControllerParametersSource=internal  P=1  I=1  D=0  N=100  b=1  c=1  InitialConditionSource=internal  InitialConditionForIntegrator=0  InitialConditionForFilter=0  ExternalReset=none  LimitOutput=off  UpperSaturationLimit=inf  LowerSaturationLimit=-inf  LinearizeAsGain=off  AntiWindupMode=none  Kb=1  TrackingMode=off  Kt=1  PParamMin=[]  PParamMax=[]  IParamMin=[]  IParamMax=[]  DParamMin=[]  DParamMax=[]  NParamMin=[]  NParamMax=[]  bParamMin=[]  bParamMax=[]  cParamMin=[]  cParamMax=[]  KbParamMin=[]  KbParamMax=[]  KtParamMin=[]  KtParamMax=[]  POutMin=[]  POutMax=[]  IOutMin=[]  IOutMax=[]  DOutMin=[]  DOutMax=[]  NOutMin=[]  NOutMax=[]  bOutMin=[]  bOutMax=[]  cOutMin=[]  cOutMax=[]  KbOutMin=[]  KbOutMax=[]  KtOutMin=[]  KtOutMax=[]  IntegratorOutMin=[]  IntegratorOutMax=[]  FilterOutMin=[]  FilterOutMax=[]  SumOutMin=[]  SumOutMax=[]  Sum1OutMin=[]  Sum1OutMax=[]  Sum2OutMin=[]  Sum2OutMax=[]  Sum3OutMin=[]  Sum3OutMax=[]  SumI1OutMin=[]  SumI1OutMax=[]  SumI2OutMin=[]  SumI2OutMax=[]  SumI3OutMin=[]  SumI3OutMax=[]  SumDOutMin=[]  SumDOutMax=[]  SaturationOutMin=[]  SaturationOutMax=[]  IntegratorContinuousStateAttributes=''  IntegratorStateMustResolveToSignalObject=off  IntegratorRTWStateStorageClass=Auto  FilterContinuousStateAttributes=''  FilterStateMustResolveToSignalObject=off  FilterRTWStateStorageClass=Auto  DifferentiatorICPrevScaledInput=0  DifferentiatorOutMin=[]  DifferentiatorOutMax=[]  FilterDiffOutCoefMin=[]  FilterDiffOutCoefMax=[]  SumDenOutMin=[]  SumDenOutMax=[]  SumNumOutMin=[]  SumNumOutMax=[]  ReciprocalOutMin=[]  ReciprocalOutMax=[]  DivideOutMin=[]  DivideOutMax=[]  TunerSelectOption=Transfer Function Based (PID Tuner App)
  cfblk8 : Delay
  cfblk9 : Delay  DelayLengthSource=Input port
      settings: InputPortMap=u0,p1
  cyemi_{592..605} (14 alike) : DataTypeConversion  OutDataTypeStr=double
  cfblk2 : Outport
  wires:
  cfblk1/1 -> cfblk2/1
  cfblk10/1 -> cyemi_603/1, cyemi_605/1
  cyemi_592/1 -> cfblk10/1
  cyemi_593/1 -> cfblk11/1
  cyemi_594/1 -> cfblk12/1
  cfblk9/1 -> cyemi_594/1
  cyemi_595/1 -> cfblk13/1
  cyemi_596/1 -> cfblk14/1
  cfblk5/1 -> cyemi_596/1
  cfblk13/1 -> cyemi_597/1
  cfblk11/1 -> cyemi_598/1
  cyemi_599/1 -> cfblk5/1
  cfblk12/1 -> cyemi_599/1
  cfblk7/1 -> cyemi_600/1
  cyemi_601/1 -> cfblk7/1
  cfblk14/1 -> cyemi_601/1
  cyemi_602/1 -> cfblk7/2
  cyemi_603/1 -> cfblk8/1
  cyemi_604/1 -> cfblk9/1
  cfblk8/1 -> cyemi_604/1
  cyemi_605/1 -> cfblk9/2
  cyemi_598/1 -> cyemi_595/1
  cyemi_597/1 -> cyemi_602/1, cyemi_593/1
  cyemi_600/1 -> cyemi_592/1

== system sampleModel2432_pp_1_2/cfblk219/cfblk11 ==
  cfblk1 : Inport
  cfblk7 : Inport  Port=2
  cfblk8 : Inport  Port=3
  Action Port : ActionPort
  cfblk3 : DiscreteTransferFcn
  cfblk4 : simulink/Discrete/Transfer Fcn First Order  PoleZ=0.95  ICPrevOutput=0.0  DoSatur=off
      settings: SourceProductName=Simulink
  cfblk5 : UnitDelay  SampleTime=-1
  cfblk6 : DiscreteStateSpace  SampleTime=-1
  cyemi_{609..612} (4 alike) : DataTypeConversion  OutDataTypeStr=double
  cfblk2 : Outport
  cfblk9 : Outport  Port=2
  cfblk10 : Outport  Port=3
  wires:
  cfblk6/1 -> cfblk9/1
  cfblk3/1 -> cfblk10/1
  cfblk5/1 -> cfblk2/1
  cyemi_609/1 -> cfblk3/1
  cfblk1/1 -> cyemi_609/1
  cyemi_610/1 -> cfblk4/1
  cfblk7/1 -> cyemi_610/1
  cyemi_611/1 -> cfblk5/1
  cfblk4/1 -> cyemi_611/1
  cyemi_612/1 -> cfblk6/1
  cfblk8/1 -> cyemi_612/1

== system sampleModel2432_pp_1_2/cfblk224/cfblk8 ==
  cfblk1 : Inport
  cfblk12 : Inport  Port=2
  cfblk13 : Inport  Port=3
  Action Port : ActionPort  ActionType=then
  cfblk10 : Delay  DelayLengthSource=Input port
      settings: InputPortMap=u0,p1
  cfblk11 : Delay  ShowEnablePort=on
      settings: InputPortMap=u0,e6
  cfblk5 : simulink/Discrete/Tapped Delay  vinit=0.0  samptime=-1  NumDelays=1  DelayOrder=Oldest  includeCurrent=off
  cfblk6 : simulink/Continuous/PID Controller  Controller=PID  TimeDomain=Discrete-time  SampleTime=-1  IntegratorMethod=Forward Euler  FilterMethod=Forward Euler  Form=Parallel  UseFilter=on  ControllerParametersSource=internal  P=1  I=1  D=0  N=100  InitialConditionSource=internal  InitialConditionForIntegrator=0  InitialConditionForFilter=0  ExternalReset=none  LimitOutput=off  UpperSaturationLimit=inf  LowerSaturationLimit=-inf  LinearizeAsGain=off  AntiWindupMode=none  Kb=1  TrackingMode=off  Kt=1  PParamMin=[]  PParamMax=[]  IParamMin=[]  IParamMax=[]  DParamMin=[]  DParamMax=[]  NParamMin=[]  NParamMax=[]  KbParamMin=[]  KbParamMax=[]  KtParamMin=[]  KtParamMax=[]  POutMin=[]  POutMax=[]  IOutMin=[]  IOutMax=[]  DOutMin=[]  DOutMax=[]  NOutMin=[]  NOutMax=[]  KbOutMin=[]  KbOutMax=[]  KtOutMin=[]  KtOutMax=[]  IntegratorOutMin=[]  IntegratorOutMax=[]  FilterOutMin=[]  FilterOutMax=[]  SumOutMin=[]  SumOutMax=[]  SumI1OutMin=[]  SumI1OutMax=[]  SumI2OutMin=[]  SumI2OutMax=[]  SumI3OutMin=[]  SumI3OutMax=[]  SumDOutMin=[]  SumDOutMax=[]  SaturationOutMin=[]  SaturationOutMax=[]  IntegratorContinuousStateAttributes=''  IntegratorStateMustResolveToSignalObject=off  IntegratorRTWStateStorageClass=Auto  FilterContinuousStateAttributes=''  FilterStateMustResolveToSignalObject=off  FilterRTWStateStorageClass=Auto  DifferentiatorICPrevScaledInput=0  DifferentiatorOutMin=[]  DifferentiatorOutMax=[]  FilterDiffOutCoefMin=[]  FilterDiffOutCoefMax=[]  SumDenOutMin=[]  SumDenOutMax=[]  SumNumOutMin=[]  SumNumOutMax=[]  ReciprocalOutMin=[]  ReciprocalOutMax=[]  DivideOutMin=[]  DivideOutMax=[]  TunerSelectOption=Transfer Function Based (PID Tuner App)
  cfblk7 : DiscreteZeroPole  Poles=[0 0.5]  Gain=1  SampleTime=-1
  cfblk8 : Delay  DelayLengthSource=Input port
      settings: InputPortMap=u0,p1
  cfblk9 : Delay  ShowEnablePort=on
      settings: InputPortMap=u0,e6
  cyemi_{672..684} (13 alike) : DataTypeConversion  OutDataTypeStr=double
  cfblk2 : Outport
  cfblk14 : Outport  Port=2
  cfblk15 : Outport  Port=3
  cfblk16 : Outport  Port=4
  wires:
  cfblk12/1 -> cfblk2/1, cyemi_680/1, cyemi_682/1
  cfblk1/1 -> cfblk14/1, cyemi_684/1
  cfblk7/1 -> cfblk16/1
  cfblk11/1 -> cyemi_678/1, cyemi_683/1
  cyemi_672/1 -> cfblk10/1
  cfblk9/1 -> cyemi_672/1
  cyemi_673/1 -> cfblk10/2
  cyemi_674/1 -> cfblk11/1
  cfblk6/1 -> cyemi_674/1, cyemi_675/1
  cyemi_675/1 -> cfblk11/2
  cfblk8/1 -> cyemi_676/1
  cfblk5/1 -> cyemi_677/1
  cyemi_678/1 -> cfblk5/1
  cyemi_679/1 -> cfblk6/1
  cfblk13/1 -> cyemi_679/1
  cyemi_680/1 -> cfblk7/1
  cyemi_681/1 -> cfblk8/1
  cfblk10/1 -> cyemi_681/1
  cyemi_682/1 -> cfblk8/2
  cyemi_683/1 -> cfblk9/1
  cyemi_684/1 -> cfblk9/2
  cyemi_676/1 -> cfblk15/1
  cyemi_677/1 -> cyemi_673/1

== system sampleModel2432_pp_1_2/cfblk224/cfblk9 ==
  cfblk1 : Inport
  cfblk8 : Inport  Port=2
  Action Port : ActionPort  ActionType=else
  cfblk10 : Delay
  cfblk4 : Delay  ShowEnablePort=on
      settings: InputPortMap=u0,e6
  cfblk5 : simulink/Continuous/PID Controller (2DOF)  Controller=PID  TimeDomain=Discrete-time  SampleTime=-1  IntegratorMethod=Forward Euler  FilterMethod=Forward Euler  Form=Parallel  UseFilter=on  ControllerParametersSource=internal  P=1  I=1  D=0  N=100  b=1  c=1  InitialConditionSource=internal  InitialConditionForIntegrator=0  InitialConditionForFilter=0  ExternalReset=none  LimitOutput=off  UpperSaturationLimit=inf  LowerSaturationLimit=-inf  LinearizeAsGain=off  AntiWindupMode=none  Kb=1  TrackingMode=off  Kt=1  PParamMin=[]  PParamMax=[]  IParamMin=[]  IParamMax=[]  DParamMin=[]  DParamMax=[]  NParamMin=[]  NParamMax=[]  bParamMin=[]  bParamMax=[]  cParamMin=[]  cParamMax=[]  KbParamMin=[]  KbParamMax=[]  KtParamMin=[]  KtParamMax=[]  POutMin=[]  POutMax=[]  IOutMin=[]  IOutMax=[]  DOutMin=[]  DOutMax=[]  NOutMin=[]  NOutMax=[]  bOutMin=[]  bOutMax=[]  cOutMin=[]  cOutMax=[]  KbOutMin=[]  KbOutMax=[]  KtOutMin=[]  KtOutMax=[]  IntegratorOutMin=[]  IntegratorOutMax=[]  FilterOutMin=[]  FilterOutMax=[]  SumOutMin=[]  SumOutMax=[]  Sum1OutMin=[]  Sum1OutMax=[]  Sum2OutMin=[]  Sum2OutMax=[]  Sum3OutMin=[]  Sum3OutMax=[]  SumI1OutMin=[]  SumI1OutMax=[]  SumI2OutMin=[]  SumI2OutMax=[]  SumI3OutMin=[]  SumI3OutMax=[]  SumDOutMin=[]  SumDOutMax=[]  SaturationOutMin=[]  SaturationOutMax=[]  IntegratorContinuousStateAttributes=''  IntegratorStateMustResolveToSignalObject=off  IntegratorRTWStateStorageClass=Auto  FilterContinuousStateAttributes=''  FilterStateMustResolveToSignalObject=off  FilterRTWStateStorageClass=Auto  DifferentiatorICPrevScaledInput=0  DifferentiatorOutMin=[]  DifferentiatorOutMax=[]  FilterDiffOutCoefMin=[]  FilterDiffOutCoefMax=[]  SumDenOutMin=[]  SumDenOutMax=[]  SumNumOutMin=[]  SumNumOutMax=[]  ReciprocalOutMin=[]  ReciprocalOutMax=[]  DivideOutMin=[]  DivideOutMax=[]  TunerSelectOption=Transfer Function Based (PID Tuner App)
  cfblk6 : DiscreteFilter
  cyemi_{687..694} (8 alike) : DataTypeConversion  OutDataTypeStr=double
  cfblk2 : Outport
  cfblk9 : Outport  Port=2
  wires:
  cfblk5/1 -> cfblk2/1
  cfblk4/1 -> cfblk9/1, cyemi_687/1
  cyemi_687/1 -> cfblk10/1
  cfblk10/1 -> cyemi_688/1
  cyemi_689/1 -> cfblk4/1
  cyemi_690/1 -> cfblk4/2
  cyemi_691/1 -> cfblk5/1
  cfblk1/1 -> cyemi_691/1
  cyemi_692/1 -> cfblk5/2
  cfblk8/1 -> cyemi_692/1
  cyemi_693/1 -> cfblk6/1
  cfblk6/1 -> cyemi_694/1
  cyemi_694/1 -> cyemi_689/1
  cyemi_688/1 -> cyemi_693/1, cyemi_690/1

== system sampleModel2432_pp_1_2/cfblk225/cfblk16 ==
  cfblk1 : Inport
  cfblk7 : Inport  Port=2
  Action Port : ActionPort
  cfblk3 : simulink/Discrete/Transfer Fcn Real Zero  ZeroZ=0.75  ICPrevInput=0.0  DoSatur=off
      settings: SourceProductName=Simulink  SourceProductBaseCode=SL
  cfblk5 : simulink/Discrete/Transfer Fcn Lead or Lag  PoleZ=0.95  ZeroZ=0.75  ICPrevOutput=0.0  ICPrevInput=0.0  DoSatur=off
      settings: SourceProductName=Simulink  SourceProductBaseCode=SL
  cfblk6 : UnitDelay  SampleTime=-1
  cyemi_{704..707} (4 alike) : DataTypeConversion  OutDataTypeStr=double
  cfblk2 : Outport
  wires:
  cyemi_704/1 -> cfblk3/1
  cfblk6/1 -> cyemi_704/1
  cfblk1/1 -> cyemi_705/1
  cyemi_706/1 -> cfblk5/1
  cfblk7/1 -> cyemi_706/1
  cyemi_707/1 -> cfblk6/1
  cfblk5/1 -> cyemi_707/1
  cyemi_705/1 -> cfblk2/1
